simulink model "TxSteering_RxMVDR_4x4_HDL_IQ"  (R2020a)
settings: Solver=FixedStepDiscrete  StartTime=0.0  StopTime=stoptime*0 + inf  RelTol=1e-3
PreLoadFcn:
  | load('iq_bus_obj.mat');
  | model_init
InitFcn:
  | model_init
model workspace (MAT data in the model file):
  socvcb : containers.Map (value not decoded)
values from neighbouring files (symbols this model uses):
  BackSubstitutePrototype = fi(0, matrixdivbacksub_dt)    [model_init.m]
  DataSampleRate = ConverterSampleRate/DecimInterpFactor    (= 245760000)    [model_init.m]
  fc = ConverterSampleRate/4    (= 491520000)    [model_init.m]
  FPGAClkRate = DataSampleRate/VectorSamplingFactor    (= 245760000)    [model_init.m]
  matrixDivDelay = NumberOfCORDICIterations*10 + 86    [model_init.m]
  movavg_bitshift = nextpow2(sqrt(windowSize))    [model_init.m]
  mvdrPipelineDelay = covMatDelay+movAvgDelay+matrixDivDelay+normResponseDelay    [model_init.m]
  NCO_bits = 14    [model_init.m]
  numArrayElements = 4    [model_init.m]
  NumberOfCORDICIterations = matrixdivin_dt.WordLength - 1    [model_init.m]
  S2MM_frame_size = FrameSize*4    (= 40000)    [host_io_init.m]    (also in model_init.m = 1000)
  windowSize = 1024    [model_init.m]
undefined symbols (not defined in the file or in its folder): Fo, Fs, N, physconst
libraries: hdlsllib x268, simulink x53, dspsolvers x1, embreciprocals x1, dsphdlsigops x1
(part 10 of 12)

== system TxSteering_RxMVDR_4x4_HDL_IQ/DUT/MVDR/Compute Weight Vector/Matrix Left Divide/CORDIC/4x4 Complex CORDIC Matrix Left Divide/Q'B, R 4x4 Complex CORDIC Systolic Array/Leading Complex Row Rotation - 2/Rotate first element to real/Q'B, R Row Rotations - Real/Same Datatype3 ==
  Data : Inport
  Reference : Inport  Port=2
  Data Type Duplicate : DataTypeDuplicate
  DataOut : Outport  VectorParamsAs1DForOutWhenUnconnected=off
  wires:
  Data/1 -> Data Type Duplicate/1, DataOut/1
  Reference/1 -> Data Type Duplicate/2

== system TxSteering_RxMVDR_4x4_HDL_IQ/DUT/MVDR/Compute Weight Vector/Matrix Left Divide/CORDIC/4x4 Complex CORDIC Matrix Left Divide/Q'B, R 4x4 Complex CORDIC Systolic Array/Leading Complex Row Rotation - 2/Rotate first element to real - 1/Q'B, R Row Rotations - Real/CORDIC Counter ==
  validIn : Inport
  Compare To Constant : simulink/Logic and Bit Operations/Compare To Constant  relop===  const=NumberOfCORDICIterations-1  OutDataTypeStr=boolean
  Compare To Zero : simulink/Logic and Bit Operations/Compare To Zero  relop=>  OutDataTypeStr=boolean
  HDL Counter1 : hdlsllib/Sources/HDL Counter  CountType=Count limited  CountInit=0  CountStep=1  CountMax=NumberOfCORDICIterations-1  CountFromType=Initial value  CountFrom=0  CountResetPort=off  CountLoadPort=off  CountEnbPort=on  CountDirPort=off  CountDataType=Unsigned  CountWordLen=nextpow2(NumberOfCORDICIterations)  CountFracLen=0  CountSampTime=1
  OR : Logic  Operator=OR  IconShape=distinctive  AllPortsSameDT=off  OutDataTypeStr=boolean
  SR_latch : Subsystem
  State Control : StateControl  StateControl=Synchronous
  ValidIn to Ready Logic : Subsystem
  count_is_positive : Outport  VectorParamsAs1DForOutWhenUnconnected=off
  count : Outport  Port=2  VectorParamsAs1DForOutWhenUnconnected=off
  last : Outport  Port=3  VectorParamsAs1DForOutWhenUnconnected=off
  ready : Outport  Port=4  VectorParamsAs1DForOutWhenUnconnected=off
  wires:
  HDL Counter1/1 -> Compare To Zero/1, count/1, Compare To Constant/1  "count"
  OR/1 -> HDL Counter1/1
  Compare To Zero/1 -> count_is_positive/1, OR/1
  Compare To Constant/1 -> SR_latch/1(S), last/1
  validIn/1 -> ValidIn to Ready Logic/2(validIn), SR_latch/2(R), OR/2
  SR_latch/1(Q) -> ValidIn to Ready Logic/1(readyIn)  "ready"
  ValidIn to Ready Logic/1(readyOut) -> ready/1

== system TxSteering_RxMVDR_4x4_HDL_IQ/DUT/MVDR/Compute Weight Vector/Matrix Left Divide/CORDIC/4x4 Complex CORDIC Matrix Left Divide/Q'B, R 4x4 Complex CORDIC Systolic Array/Leading Complex Row Rotation - 2/Rotate first element to real - 1/Q'B, R Row Rotations - Real/Same Datatype ==
  Data : Inport
  Reference : Inport  Port=2
  Data Type Duplicate : DataTypeDuplicate
  DataOut : Outport  VectorParamsAs1DForOutWhenUnconnected=off
  wires:
  Data/1 -> Data Type Duplicate/1, DataOut/1
  Reference/1 -> Data Type Duplicate/2

== system TxSteering_RxMVDR_4x4_HDL_IQ/DUT/MVDR/Compute Weight Vector/Matrix Left Divide/CORDIC/4x4 Complex CORDIC Matrix Left Divide/Q'B, R 4x4 Complex CORDIC Systolic Array/Leading Complex Row Rotation - 2/Rotate first element to real - 1/Q'B, R Row Rotations - Real/Same Datatype1 ==
  Data : Inport
  Reference : Inport  Port=2
  Data Type Duplicate : DataTypeDuplicate
  DataOut : Outport  VectorParamsAs1DForOutWhenUnconnected=off
  wires:
  Data/1 -> Data Type Duplicate/1, DataOut/1
  Reference/1 -> Data Type Duplicate/2

== system TxSteering_RxMVDR_4x4_HDL_IQ/DUT/MVDR/Compute Weight Vector/Matrix Left Divide/CORDIC/4x4 Complex CORDIC Matrix Left Divide/Q'B, R 4x4 Complex CORDIC Systolic Array/Leading Complex Row Rotation - 2/Rotate first element to real - 1/Q'B, R Row Rotations - Real/Same Datatype2 ==
  Data : Inport
  Reference : Inport  Port=2
  Data Type Duplicate : DataTypeDuplicate
  DataOut : Outport  VectorParamsAs1DForOutWhenUnconnected=off
  wires:
  Data/1 -> Data Type Duplicate/1, DataOut/1
  Reference/1 -> Data Type Duplicate/2

== system TxSteering_RxMVDR_4x4_HDL_IQ/DUT/MVDR/Compute Weight Vector/Matrix Left Divide/CORDIC/4x4 Complex CORDIC Matrix Left Divide/Q'B, R 4x4 Complex CORDIC Systolic Array/Leading Complex Row Rotation - 2/Rotate first element to real - 1/Q'B, R Row Rotations - Real/Same Datatype3 ==
  Data : Inport
  Reference : Inport  Port=2
  Data Type Duplicate : DataTypeDuplicate
  DataOut : Outport  VectorParamsAs1DForOutWhenUnconnected=off
  wires:
  Data/1 -> Data Type Duplicate/1, DataOut/1
  Reference/1 -> Data Type Duplicate/2

== system TxSteering_RxMVDR_4x4_HDL_IQ/DUT/MVDR/Compute Weight Vector/Matrix Left Divide/CORDIC/4x4 Complex CORDIC Matrix Left Divide/Q'B, R 4x4 Complex CORDIC Systolic Array/Leading Complex Row Rotation - 3/Q'B, R Row Rotations - Complex/CORDIC Counter/SR_latch ==
  S : Inport
  R : Inport  Port=2
  AND : Logic  IconShape=distinctive  AllPortsSameDT=off  OutDataTypeStr=boolean
  NOT : Logic  Operator=NOT  IconShape=distinctive  AllPortsSameDT=off  OutDataTypeStr=boolean
  OR : Logic  Operator=OR  IconShape=distinctive  AllPortsSameDT=off  OutDataTypeStr=boolean
  Prev : UnitDelay  InitialCondition=1  SampleTime=-1  HasFrameUpgradeWarning=on
  Q : Outport  VectorParamsAs1DForOutWhenUnconnected=off
  wires:
  R/1 -> NOT/1
  NOT/1 -> AND/1
  AND/1 -> OR/2
  Prev/1 -> Q/1, AND/2
  OR/1 -> Prev/1
  S/1 -> OR/1

== system TxSteering_RxMVDR_4x4_HDL_IQ/DUT/MVDR/Compute Weight Vector/Matrix Left Divide/CORDIC/4x4 Complex CORDIC Matrix Left Divide/Q'B, R 4x4 Complex CORDIC Systolic Array/Leading Complex Row Rotation - 3/Q'B, R Row Rotations - Complex/CORDIC Counter/ValidIn to Ready Logic ==
  readyIn : Inport
  validIn : Inport  Port=2
  AND : Logic  IconShape=distinctive  AllPortsSameDT=off  OutDataTypeStr=boolean
  NOT : Logic  Operator=NOT  IconShape=distinctive  AllPortsSameDT=off  OutDataTypeStr=boolean
  readyOut : Outport  VectorParamsAs1DForOutWhenUnconnected=off
  wires:
  validIn/1 -> NOT/1
  readyIn/1 -> AND/1
  AND/1 -> readyOut/1
  NOT/1 -> AND/2

== system TxSteering_RxMVDR_4x4_HDL_IQ/DUT/MVDR/Compute Weight Vector/Matrix Left Divide/CORDIC/4x4 Complex CORDIC Matrix Left Divide/Q'B, R 4x4 Complex CORDIC Systolic Array/Leading Complex Row Rotation - 3/Rotate first element to real/Q'B, R Row Rotations - Real/CORDIC Counter ==
  validIn : Inport
  Compare To Constant : simulink/Logic and Bit Operations/Compare To Constant  relop===  const=NumberOfCORDICIterations-1  OutDataTypeStr=boolean
  Compare To Zero : simulink/Logic and Bit Operations/Compare To Zero  relop=>  OutDataTypeStr=boolean
  HDL Counter1 : hdlsllib/Sources/HDL Counter  CountType=Count limited  CountInit=0  CountStep=1  CountMax=NumberOfCORDICIterations-1  CountFromType=Initial value  CountFrom=0  CountResetPort=off  CountLoadPort=off  CountEnbPort=on  CountDirPort=off  CountDataType=Unsigned  CountWordLen=nextpow2(NumberOfCORDICIterations)  CountFracLen=0  CountSampTime=1
  OR : Logic  Operator=OR  IconShape=distinctive  AllPortsSameDT=off  OutDataTypeStr=boolean
  SR_latch : Subsystem
  State Control : StateControl  StateControl=Synchronous
  ValidIn to Ready Logic : Subsystem
  count_is_positive : Outport  VectorParamsAs1DForOutWhenUnconnected=off
  count : Outport  Port=2  VectorParamsAs1DForOutWhenUnconnected=off
  last : Outport  Port=3  VectorParamsAs1DForOutWhenUnconnected=off
  ready : Outport  Port=4  VectorParamsAs1DForOutWhenUnconnected=off
  wires:
  HDL Counter1/1 -> Compare To Zero/1, count/1, Compare To Constant/1  "count"
  OR/1 -> HDL Counter1/1
  Compare To Zero/1 -> count_is_positive/1, OR/1
  Compare To Constant/1 -> SR_latch/1(S), last/1
  validIn/1 -> ValidIn to Ready Logic/2(validIn), SR_latch/2(R), OR/2
  SR_latch/1(Q) -> ValidIn to Ready Logic/1(readyIn)  "ready"
  ValidIn to Ready Logic/1(readyOut) -> ready/1

== system TxSteering_RxMVDR_4x4_HDL_IQ/DUT/MVDR/Compute Weight Vector/Matrix Left Divide/CORDIC/4x4 Complex CORDIC Matrix Left Divide/Q'B, R 4x4 Complex CORDIC Systolic Array/Leading Complex Row Rotation - 3/Rotate first element to real/Q'B, R Row Rotations - Real/Same Datatype ==
  Data : Inport
  Reference : Inport  Port=2
  Data Type Duplicate : DataTypeDuplicate
  DataOut : Outport  VectorParamsAs1DForOutWhenUnconnected=off
  wires:
  Data/1 -> Data Type Duplicate/1, DataOut/1
  Reference/1 -> Data Type Duplicate/2

== system TxSteering_RxMVDR_4x4_HDL_IQ/DUT/MVDR/Compute Weight Vector/Matrix Left Divide/CORDIC/4x4 Complex CORDIC Matrix Left Divide/Q'B, R 4x4 Complex CORDIC Systolic Array/Leading Complex Row Rotation - 3/Rotate first element to real/Q'B, R Row Rotations - Real/Same Datatype1 ==
  Data : Inport
  Reference : Inport  Port=2
  Data Type Duplicate : DataTypeDuplicate
  DataOut : Outport  VectorParamsAs1DForOutWhenUnconnected=off
  wires:
  Data/1 -> Data Type Duplicate/1, DataOut/1
  Reference/1 -> Data Type Duplicate/2

== system TxSteering_RxMVDR_4x4_HDL_IQ/DUT/MVDR/Compute Weight Vector/Matrix Left Divide/CORDIC/4x4 Complex CORDIC Matrix Left Divide/Q'B, R 4x4 Complex CORDIC Systolic Array/Leading Complex Row Rotation - 3/Rotate first element to real/Q'B, R Row Rotations - Real/Same Datatype2 ==
  Data : Inport
  Reference : Inport  Port=2
  Data Type Duplicate : DataTypeDuplicate
  DataOut : Outport  VectorParamsAs1DForOutWhenUnconnected=off
  wires:
  Data/1 -> Data Type Duplicate/1, DataOut/1
  Reference/1 -> Data Type Duplicate/2

== system TxSteering_RxMVDR_4x4_HDL_IQ/DUT/MVDR/Compute Weight Vector/Matrix Left Divide/CORDIC/4x4 Complex CORDIC Matrix Left Divide/Q'B, R 4x4 Complex CORDIC Systolic Array/Leading Complex Row Rotation - 3/Rotate first element to real/Q'B, R Row Rotations - Real/Same Datatype3 ==
  Data : Inport
  Reference : Inport  Port=2
  Data Type Duplicate : DataTypeDuplicate
  DataOut : Outport  VectorParamsAs1DForOutWhenUnconnected=off
  wires:
  Data/1 -> Data Type Duplicate/1, DataOut/1
  Reference/1 -> Data Type Duplicate/2

== system TxSteering_RxMVDR_4x4_HDL_IQ/DUT/MVDR/Compute Weight Vector/Matrix Left Divide/CORDIC/4x4 Complex CORDIC Matrix Left Divide/Q'B, R 4x4 Complex CORDIC Systolic Array/Leading Complex Row Rotation - 3/Rotate first element to real - 1/Q'B, R Row Rotations - Real/CORDIC Counter ==
  validIn : Inport
  Compare To Constant : simulink/Logic and Bit Operations/Compare To Constant  relop===  const=NumberOfCORDICIterations-1  OutDataTypeStr=boolean
  Compare To Zero : simulink/Logic and Bit Operations/Compare To Zero  relop=>  OutDataTypeStr=boolean
  HDL Counter1 : hdlsllib/Sources/HDL Counter  CountType=Count limited  CountInit=0  CountStep=1  CountMax=NumberOfCORDICIterations-1  CountFromType=Initial value  CountFrom=0  CountResetPort=off  CountLoadPort=off  CountEnbPort=on  CountDirPort=off  CountDataType=Unsigned  CountWordLen=nextpow2(NumberOfCORDICIterations)  CountFracLen=0  CountSampTime=1
  OR : Logic  Operator=OR  IconShape=distinctive  AllPortsSameDT=off  OutDataTypeStr=boolean
  SR_latch : Subsystem
  State Control : StateControl  StateControl=Synchronous
  ValidIn to Ready Logic : Subsystem
  count_is_positive : Outport  VectorParamsAs1DForOutWhenUnconnected=off
  count : Outport  Port=2  VectorParamsAs1DForOutWhenUnconnected=off
  last : Outport  Port=3  VectorParamsAs1DForOutWhenUnconnected=off
  ready : Outport  Port=4  VectorParamsAs1DForOutWhenUnconnected=off
  wires:
  ValidIn to Ready Logic/1(readyOut) -> ready/1
  SR_latch/1(Q) -> ValidIn to Ready Logic/1(readyIn)  "ready"
  validIn/1 -> OR/2, SR_latch/2(R), ValidIn to Ready Logic/2(validIn)
  Compare To Constant/1 -> last/1, SR_latch/1(S)
  Compare To Zero/1 -> OR/1, count_is_positive/1
  OR/1 -> HDL Counter1/1
  HDL Counter1/1 -> Compare To Constant/1, count/1, Compare To Zero/1  "count"

== system TxSteering_RxMVDR_4x4_HDL_IQ/DUT/MVDR/Compute Weight Vector/Matrix Left Divide/CORDIC/4x4 Complex CORDIC Matrix Left Divide/Q'B, R 4x4 Complex CORDIC Systolic Array/Leading Complex Row Rotation - 3/Rotate first element to real - 1/Q'B, R Row Rotations - Real/Same Datatype ==
  Data : Inport
  Reference : Inport  Port=2
  Data Type Duplicate : DataTypeDuplicate
  DataOut : Outport  VectorParamsAs1DForOutWhenUnconnected=off
  wires:
  Data/1 -> Data Type Duplicate/1, DataOut/1
  Reference/1 -> Data Type Duplicate/2

== system TxSteering_RxMVDR_4x4_HDL_IQ/DUT/MVDR/Compute Weight Vector/Matrix Left Divide/CORDIC/4x4 Complex CORDIC Matrix Left Divide/Q'B, R 4x4 Complex CORDIC Systolic Array/Leading Complex Row Rotation - 3/Rotate first element to real - 1/Q'B, R Row Rotations - Real/Same Datatype1 ==
  Data : Inport
  Reference : Inport  Port=2
  Data Type Duplicate : DataTypeDuplicate
  DataOut : Outport  VectorParamsAs1DForOutWhenUnconnected=off
  wires:
  Data/1 -> Data Type Duplicate/1, DataOut/1
  Reference/1 -> Data Type Duplicate/2

== system TxSteering_RxMVDR_4x4_HDL_IQ/DUT/MVDR/Compute Weight Vector/Matrix Left Divide/CORDIC/4x4 Complex CORDIC Matrix Left Divide/Q'B, R 4x4 Complex CORDIC Systolic Array/Leading Complex Row Rotation - 3/Rotate first element to real - 1/Q'B, R Row Rotations - Real/Same Datatype2 ==
  Data : Inport
  Reference : Inport  Port=2
  Data Type Duplicate : DataTypeDuplicate
  DataOut : Outport  VectorParamsAs1DForOutWhenUnconnected=off
  wires:
  Data/1 -> Data Type Duplicate/1, DataOut/1
  Reference/1 -> Data Type Duplicate/2

== system TxSteering_RxMVDR_4x4_HDL_IQ/DUT/MVDR/Compute Weight Vector/Matrix Left Divide/CORDIC/4x4 Complex CORDIC Matrix Left Divide/Q'B, R 4x4 Complex CORDIC Systolic Array/Leading Complex Row Rotation - 3/Rotate first element to real - 1/Q'B, R Row Rotations - Real/Same Datatype3 ==
  Data : Inport
  Reference : Inport  Port=2
  Data Type Duplicate : DataTypeDuplicate
  DataOut : Outport  VectorParamsAs1DForOutWhenUnconnected=off
  wires:
  Data/1 -> Data Type Duplicate/1, DataOut/1
  Reference/1 -> Data Type Duplicate/2

== system TxSteering_RxMVDR_4x4_HDL_IQ/DUT/MVDR/Compute Weight Vector/Matrix Left Divide/CORDIC/4x4 Complex CORDIC Matrix Left Divide/Q'B, R 4x4 Complex CORDIC Systolic Array/Leading Complex Row Rotation - 4/Q'B, R Row Rotations - Complex/CORDIC Counter/SR_latch ==
  S : Inport
  R : Inport  Port=2
  AND : Logic  IconShape=distinctive  AllPortsSameDT=off  OutDataTypeStr=boolean
  NOT : Logic  Operator=NOT  IconShape=distinctive  AllPortsSameDT=off  OutDataTypeStr=boolean
  OR : Logic  Operator=OR  IconShape=distinctive  AllPortsSameDT=off  OutDataTypeStr=boolean
  Prev : UnitDelay  InitialCondition=1  SampleTime=-1  HasFrameUpgradeWarning=on
  Q : Outport  VectorParamsAs1DForOutWhenUnconnected=off
  wires:
  R/1 -> NOT/1
  NOT/1 -> AND/1
  AND/1 -> OR/2
  Prev/1 -> Q/1, AND/2
  OR/1 -> Prev/1
  S/1 -> OR/1

== system TxSteering_RxMVDR_4x4_HDL_IQ/DUT/MVDR/Compute Weight Vector/Matrix Left Divide/CORDIC/4x4 Complex CORDIC Matrix Left Divide/Q'B, R 4x4 Complex CORDIC Systolic Array/Leading Complex Row Rotation - 4/Q'B, R Row Rotations - Complex/CORDIC Counter/ValidIn to Ready Logic ==
  readyIn : Inport
  validIn : Inport  Port=2
  AND : Logic  IconShape=distinctive  AllPortsSameDT=off  OutDataTypeStr=boolean
  NOT : Logic  Operator=NOT  IconShape=distinctive  AllPortsSameDT=off  OutDataTypeStr=boolean
  readyOut : Outport  VectorParamsAs1DForOutWhenUnconnected=off
  wires:
  validIn/1 -> NOT/1
  readyIn/1 -> AND/1
  AND/1 -> readyOut/1
  NOT/1 -> AND/2

== system TxSteering_RxMVDR_4x4_HDL_IQ/DUT/MVDR/Compute Weight Vector/Matrix Left Divide/CORDIC/4x4 Complex CORDIC Matrix Left Divide/Q'B, R 4x4 Complex CORDIC Systolic Array/Leading Complex Row Rotation - 4/Rotate first element to real/Q'B, R Row Rotations - Real/CORDIC Counter ==
  validIn : Inport
  Compare To Constant : simulink/Logic and Bit Operations/Compare To Constant  relop===  const=NumberOfCORDICIterations-1  OutDataTypeStr=boolean
  Compare To Zero : simulink/Logic and Bit Operations/Compare To Zero  relop=>  OutDataTypeStr=boolean
  HDL Counter1 : hdlsllib/Sources/HDL Counter  CountType=Count limited  CountInit=0  CountStep=1  CountMax=NumberOfCORDICIterations-1  CountFromType=Initial value  CountFrom=0  CountResetPort=off  CountLoadPort=off  CountEnbPort=on  CountDirPort=off  CountDataType=Unsigned  CountWordLen=nextpow2(NumberOfCORDICIterations)  CountFracLen=0  CountSampTime=1
  OR : Logic  Operator=OR  IconShape=distinctive  AllPortsSameDT=off  OutDataTypeStr=boolean
  SR_latch : Subsystem
  State Control : StateControl  StateControl=Synchronous
  ValidIn to Ready Logic : Subsystem
  count_is_positive : Outport  VectorParamsAs1DForOutWhenUnconnected=off
  count : Outport  Port=2  VectorParamsAs1DForOutWhenUnconnected=off
  last : Outport  Port=3  VectorParamsAs1DForOutWhenUnconnected=off
  ready : Outport  Port=4  VectorParamsAs1DForOutWhenUnconnected=off
  wires:
  HDL Counter1/1 -> Compare To Zero/1, count/1, Compare To Constant/1  "count"
  OR/1 -> HDL Counter1/1
  Compare To Zero/1 -> count_is_positive/1, OR/1
  Compare To Constant/1 -> SR_latch/1(S), last/1
  validIn/1 -> ValidIn to Ready Logic/2(validIn), SR_latch/2(R), OR/2
  SR_latch/1(Q) -> ValidIn to Ready Logic/1(readyIn)  "ready"
  ValidIn to Ready Logic/1(readyOut) -> ready/1

== system TxSteering_RxMVDR_4x4_HDL_IQ/DUT/MVDR/Compute Weight Vector/Matrix Left Divide/CORDIC/4x4 Complex CORDIC Matrix Left Divide/Q'B, R 4x4 Complex CORDIC Systolic Array/Leading Complex Row Rotation - 4/Rotate first element to real/Q'B, R Row Rotations - Real/Same Datatype ==
  Data : Inport
  Reference : Inport  Port=2
  Data Type Duplicate : DataTypeDuplicate
  DataOut : Outport  VectorParamsAs1DForOutWhenUnconnected=off
  wires:
  Data/1 -> Data Type Duplicate/1, DataOut/1
  Reference/1 -> Data Type Duplicate/2

== system TxSteering_RxMVDR_4x4_HDL_IQ/DUT/MVDR/Compute Weight Vector/Matrix Left Divide/CORDIC/4x4 Complex CORDIC Matrix Left Divide/Q'B, R 4x4 Complex CORDIC Systolic Array/Leading Complex Row Rotation - 4/Rotate first element to real/Q'B, R Row Rotations - Real/Same Datatype1 ==
  Data : Inport
  Reference : Inport  Port=2
  Data Type Duplicate : DataTypeDuplicate
  DataOut : Outport  VectorParamsAs1DForOutWhenUnconnected=off
  wires:
  Data/1 -> Data Type Duplicate/1, DataOut/1
  Reference/1 -> Data Type Duplicate/2

== system TxSteering_RxMVDR_4x4_HDL_IQ/DUT/MVDR/Compute Weight Vector/Matrix Left Divide/CORDIC/4x4 Complex CORDIC Matrix Left Divide/Q'B, R 4x4 Complex CORDIC Systolic Array/Leading Complex Row Rotation - 4/Rotate first element to real/Q'B, R Row Rotations - Real/Same Datatype2 ==
  Data : Inport
  Reference : Inport  Port=2
  Data Type Duplicate : DataTypeDuplicate
  DataOut : Outport  VectorParamsAs1DForOutWhenUnconnected=off
  wires:
  Data/1 -> Data Type Duplicate/1, DataOut/1
  Reference/1 -> Data Type Duplicate/2

== system TxSteering_RxMVDR_4x4_HDL_IQ/DUT/MVDR/Compute Weight Vector/Matrix Left Divide/CORDIC/4x4 Complex CORDIC Matrix Left Divide/Q'B, R 4x4 Complex CORDIC Systolic Array/Leading Complex Row Rotation - 4/Rotate first element to real/Q'B, R Row Rotations - Real/Same Datatype3 ==
  Data : Inport
  Reference : Inport  Port=2
  Data Type Duplicate : DataTypeDuplicate
  DataOut : Outport  VectorParamsAs1DForOutWhenUnconnected=off
  wires:
  Data/1 -> Data Type Duplicate/1, DataOut/1
  Reference/1 -> Data Type Duplicate/2

== system TxSteering_RxMVDR_4x4_HDL_IQ/DUT/MVDR/Compute Weight Vector/Matrix Left Divide/CORDIC/4x4 Complex CORDIC Matrix Left Divide/Q'B, R 4x4 Complex CORDIC Systolic Array/Leading Complex Row Rotation - 4/Rotate first element to real - 1/Q'B, R Row Rotations - Real/CORDIC Counter ==
  validIn : Inport
  Compare To Constant : simulink/Logic and Bit Operations/Compare To Constant  relop===  const=NumberOfCORDICIterations-1  OutDataTypeStr=boolean
  Compare To Zero : simulink/Logic and Bit Operations/Compare To Zero  relop=>  OutDataTypeStr=boolean
  HDL Counter1 : hdlsllib/Sources/HDL Counter  CountType=Count limited  CountInit=0  CountStep=1  CountMax=NumberOfCORDICIterations-1  CountFromType=Initial value  CountFrom=0  CountResetPort=off  CountLoadPort=off  CountEnbPort=on  CountDirPort=off  CountDataType=Unsigned  CountWordLen=nextpow2(NumberOfCORDICIterations)  CountFracLen=0  CountSampTime=1
  OR : Logic  Operator=OR  IconShape=distinctive  AllPortsSameDT=off  OutDataTypeStr=boolean
  SR_latch : Subsystem
  State Control : StateControl  StateControl=Synchronous
  ValidIn to Ready Logic : Subsystem
  count_is_positive : Outport  VectorParamsAs1DForOutWhenUnconnected=off
  count : Outport  Port=2  VectorParamsAs1DForOutWhenUnconnected=off
  last : Outport  Port=3  VectorParamsAs1DForOutWhenUnconnected=off
  ready : Outport  Port=4  VectorParamsAs1DForOutWhenUnconnected=off
  wires:
  ValidIn to Ready Logic/1(readyOut) -> ready/1
  SR_latch/1(Q) -> ValidIn to Ready Logic/1(readyIn)  "ready"
  validIn/1 -> OR/2, SR_latch/2(R), ValidIn to Ready Logic/2(validIn)
  Compare To Constant/1 -> last/1, SR_latch/1(S)
  Compare To Zero/1 -> OR/1, count_is_positive/1
  OR/1 -> HDL Counter1/1
  HDL Counter1/1 -> Compare To Constant/1, count/1, Compare To Zero/1  "count"

== system TxSteering_RxMVDR_4x4_HDL_IQ/DUT/MVDR/Compute Weight Vector/Matrix Left Divide/CORDIC/4x4 Complex CORDIC Matrix Left Divide/Q'B, R 4x4 Complex CORDIC Systolic Array/Leading Complex Row Rotation - 4/Rotate first element to real - 1/Q'B, R Row Rotations - Real/Same Datatype ==
  Data : Inport
  Reference : Inport  Port=2
  Data Type Duplicate : DataTypeDuplicate
  DataOut : Outport  VectorParamsAs1DForOutWhenUnconnected=off
  wires:
  Data/1 -> Data Type Duplicate/1, DataOut/1
  Reference/1 -> Data Type Duplicate/2

== system TxSteering_RxMVDR_4x4_HDL_IQ/DUT/MVDR/Compute Weight Vector/Matrix Left Divide/CORDIC/4x4 Complex CORDIC Matrix Left Divide/Q'B, R 4x4 Complex CORDIC Systolic Array/Leading Complex Row Rotation - 4/Rotate first element to real - 1/Q'B, R Row Rotations - Real/Same Datatype1 ==
  Data : Inport
  Reference : Inport  Port=2
  Data Type Duplicate : DataTypeDuplicate
  DataOut : Outport  VectorParamsAs1DForOutWhenUnconnected=off
  wires:
  Data/1 -> Data Type Duplicate/1, DataOut/1
  Reference/1 -> Data Type Duplicate/2

== system TxSteering_RxMVDR_4x4_HDL_IQ/DUT/MVDR/Compute Weight Vector/Matrix Left Divide/CORDIC/4x4 Complex CORDIC Matrix Left Divide/Q'B, R 4x4 Complex CORDIC Systolic Array/Leading Complex Row Rotation - 4/Rotate first element to real - 1/Q'B, R Row Rotations - Real/Same Datatype2 ==
  Data : Inport
  Reference : Inport  Port=2
  Data Type Duplicate : DataTypeDuplicate
  DataOut : Outport  VectorParamsAs1DForOutWhenUnconnected=off
  wires:
  Data/1 -> Data Type Duplicate/1, DataOut/1
  Reference/1 -> Data Type Duplicate/2

== system TxSteering_RxMVDR_4x4_HDL_IQ/DUT/MVDR/Compute Weight Vector/Matrix Left Divide/CORDIC/4x4 Complex CORDIC Matrix Left Divide/Q'B, R 4x4 Complex CORDIC Systolic Array/Leading Complex Row Rotation - 4/Rotate first element to real - 1/Q'B, R Row Rotations - Real/Same Datatype3 ==
  Data : Inport
  Reference : Inport  Port=2
  Data Type Duplicate : DataTypeDuplicate
  DataOut : Outport  VectorParamsAs1DForOutWhenUnconnected=off
  wires:
  Data/1 -> Data Type Duplicate/1, DataOut/1
  Reference/1 -> Data Type Duplicate/2

== system TxSteering_RxMVDR_4x4_HDL_IQ/DUT/MVDR/Compute Weight Vector/Matrix Left Divide/CORDIC/4x4 Complex CORDIC Matrix Left Divide/Q'B, R 4x4 Complex CORDIC Systolic Array/Rotate first element to real/Q'B, R Row Rotations - Real/CORDIC Counter/SR_latch ==
  S : Inport
  R : Inport  Port=2
  AND : Logic  IconShape=distinctive  AllPortsSameDT=off  OutDataTypeStr=boolean
  NOT : Logic  Operator=NOT  IconShape=distinctive  AllPortsSameDT=off  OutDataTypeStr=boolean
  OR : Logic  Operator=OR  IconShape=distinctive  AllPortsSameDT=off  OutDataTypeStr=boolean
  Prev : UnitDelay  InitialCondition=1  SampleTime=-1  HasFrameUpgradeWarning=on
  Q : Outport  VectorParamsAs1DForOutWhenUnconnected=off
  wires:
  R/1 -> NOT/1
  NOT/1 -> AND/1
  AND/1 -> OR/2
  Prev/1 -> Q/1, AND/2
  OR/1 -> Prev/1
  S/1 -> OR/1

== system TxSteering_RxMVDR_4x4_HDL_IQ/DUT/MVDR/Compute Weight Vector/Matrix Left Divide/CORDIC/4x4 Complex CORDIC Matrix Left Divide/Q'B, R 4x4 Complex CORDIC Systolic Array/Rotate first element to real/Q'B, R Row Rotations - Real/CORDIC Counter/ValidIn to Ready Logic ==
  readyIn : Inport
  validIn : Inport  Port=2
  AND : Logic  IconShape=distinctive  AllPortsSameDT=off  OutDataTypeStr=boolean
  NOT : Logic  Operator=NOT  IconShape=distinctive  AllPortsSameDT=off  OutDataTypeStr=boolean
  readyOut : Outport  VectorParamsAs1DForOutWhenUnconnected=off
  wires:
  validIn/1 -> NOT/1
  readyIn/1 -> AND/1
  AND/1 -> readyOut/1
  NOT/1 -> AND/2

== system TxSteering_RxMVDR_4x4_HDL_IQ/DUT/MVDR/Compute Weight Vector/Matrix Left Divide/CORDIC/4x4 Complex CORDIC Matrix Left Divide/Back Substitute 4x4 Complex CORDIC/Invert first element - Folded/CORDIC Reciprocal Normalized, Folded/CORDIC Reciprocal Rotations- Folded/CORDIC Counter/SR_latch ==
  S : Inport
  R : Inport  Port=2
  AND : Logic  IconShape=distinctive  AllPortsSameDT=off  OutDataTypeStr=boolean
  NOT : Logic  Operator=NOT  IconShape=distinctive  AllPortsSameDT=off  OutDataTypeStr=boolean
  OR : Logic  Operator=OR  IconShape=distinctive  AllPortsSameDT=off  OutDataTypeStr=boolean
  Prev : UnitDelay  InitialCondition=1  SampleTime=-1  HasFrameUpgradeWarning=on
  Q : Outport  VectorParamsAs1DForOutWhenUnconnected=off
  wires:
  S/1 -> OR/1
  OR/1 -> Prev/1
  Prev/1 -> AND/2, Q/1
  AND/1 -> OR/2
  NOT/1 -> AND/1
  R/1 -> NOT/1

== system TxSteering_RxMVDR_4x4_HDL_IQ/DUT/MVDR/Compute Weight Vector/Matrix Left Divide/CORDIC/4x4 Complex CORDIC Matrix Left Divide/Back Substitute 4x4 Complex CORDIC/Invert first element - Folded/CORDIC Reciprocal Normalized, Folded/CORDIC Reciprocal Rotations- Folded/CORDIC Counter/ValidIn to Ready Logic ==
  readyIn : Inport
  validIn : Inport  Port=2
  AND : Logic  IconShape=distinctive  AllPortsSameDT=off  OutDataTypeStr=boolean
  NOT : Logic  Operator=NOT  IconShape=distinctive  AllPortsSameDT=off  OutDataTypeStr=boolean
  readyOut : Outport  VectorParamsAs1DForOutWhenUnconnected=off
  wires:
  validIn/1 -> NOT/1
  readyIn/1 -> AND/1
  AND/1 -> readyOut/1
  NOT/1 -> AND/2

== system TxSteering_RxMVDR_4x4_HDL_IQ/DUT/MVDR/Compute Weight Vector/Matrix Left Divide/CORDIC/4x4 Complex CORDIC Matrix Left Divide/Back Substitute 4x4 Complex CORDIC/Invert first element - Folded1/CORDIC Reciprocal Normalized, Folded/CORDIC Reciprocal Rotations- Folded/CORDIC Counter/SR_latch ==
  S : Inport
  R : Inport  Port=2
  AND : Logic  IconShape=distinctive  AllPortsSameDT=off  OutDataTypeStr=boolean
  NOT : Logic  Operator=NOT  IconShape=distinctive  AllPortsSameDT=off  OutDataTypeStr=boolean
  OR : Logic  Operator=OR  IconShape=distinctive  AllPortsSameDT=off  OutDataTypeStr=boolean
  Prev : UnitDelay  InitialCondition=1  SampleTime=-1  HasFrameUpgradeWarning=on
  Q : Outport  VectorParamsAs1DForOutWhenUnconnected=off
  wires:
  R/1 -> NOT/1
  NOT/1 -> AND/1
  AND/1 -> OR/2
  Prev/1 -> Q/1, AND/2
  OR/1 -> Prev/1
  S/1 -> OR/1

== system TxSteering_RxMVDR_4x4_HDL_IQ/DUT/MVDR/Compute Weight Vector/Matrix Left Divide/CORDIC/4x4 Complex CORDIC Matrix Left Divide/Back Substitute 4x4 Complex CORDIC/Invert first element - Folded1/CORDIC Reciprocal Normalized, Folded/CORDIC Reciprocal Rotations- Folded/CORDIC Counter/ValidIn to Ready Logic ==
  readyIn : Inport
  validIn : Inport  Port=2
  AND : Logic  IconShape=distinctive  AllPortsSameDT=off  OutDataTypeStr=boolean
  NOT : Logic  Operator=NOT  IconShape=distinctive  AllPortsSameDT=off  OutDataTypeStr=boolean
  readyOut : Outport  VectorParamsAs1DForOutWhenUnconnected=off
  wires:
  validIn/1 -> NOT/1
  readyIn/1 -> AND/1
  AND/1 -> readyOut/1
  NOT/1 -> AND/2

== system TxSteering_RxMVDR_4x4_HDL_IQ/DUT/MVDR/Compute Weight Vector/Matrix Left Divide/CORDIC/4x4 Complex CORDIC Matrix Left Divide/Back Substitute 4x4 Complex CORDIC/Invert first element - Folded2/CORDIC Reciprocal Normalized, Folded/CORDIC Reciprocal Rotations- Folded/CORDIC Counter/SR_latch ==
  S : Inport
  R : Inport  Port=2
  AND : Logic  IconShape=distinctive  AllPortsSameDT=off  OutDataTypeStr=boolean
  NOT : Logic  Operator=NOT  IconShape=distinctive  AllPortsSameDT=off  OutDataTypeStr=boolean
  OR : Logic  Operator=OR  IconShape=distinctive  AllPortsSameDT=off  OutDataTypeStr=boolean
  Prev : UnitDelay  InitialCondition=1  SampleTime=-1  HasFrameUpgradeWarning=on
  Q : Outport  VectorParamsAs1DForOutWhenUnconnected=off
  wires:
  R/1 -> NOT/1
  NOT/1 -> AND/1
  AND/1 -> OR/2
  Prev/1 -> Q/1, AND/2
  OR/1 -> Prev/1
  S/1 -> OR/1

== system TxSteering_RxMVDR_4x4_HDL_IQ/DUT/MVDR/Compute Weight Vector/Matrix Left Divide/CORDIC/4x4 Complex CORDIC Matrix Left Divide/Back Substitute 4x4 Complex CORDIC/Invert first element - Folded2/CORDIC Reciprocal Normalized, Folded/CORDIC Reciprocal Rotations- Folded/CORDIC Counter/ValidIn to Ready Logic ==
  readyIn : Inport
  validIn : Inport  Port=2
  AND : Logic  IconShape=distinctive  AllPortsSameDT=off  OutDataTypeStr=boolean
  NOT : Logic  Operator=NOT  IconShape=distinctive  AllPortsSameDT=off  OutDataTypeStr=boolean
  readyOut : Outport  VectorParamsAs1DForOutWhenUnconnected=off
  wires:
  validIn/1 -> NOT/1
  readyIn/1 -> AND/1
  AND/1 -> readyOut/1
  NOT/1 -> AND/2

== system TxSteering_RxMVDR_4x4_HDL_IQ/DUT/MVDR/Compute Weight Vector/Matrix Left Divide/CORDIC/4x4 Complex CORDIC Matrix Left Divide/Back Substitute 4x4 Complex CORDIC/Invert first element - Folded3/CORDIC Reciprocal Normalized, Folded/CORDIC Reciprocal Rotations- Folded/CORDIC Counter/SR_latch ==
  S : Inport
  R : Inport  Port=2
  AND : Logic  IconShape=distinctive  AllPortsSameDT=off  OutDataTypeStr=boolean
  NOT : Logic  Operator=NOT  IconShape=distinctive  AllPortsSameDT=off  OutDataTypeStr=boolean
  OR : Logic  Operator=OR  IconShape=distinctive  AllPortsSameDT=off  OutDataTypeStr=boolean
  Prev : UnitDelay  InitialCondition=1  SampleTime=-1  HasFrameUpgradeWarning=on
  Q : Outport  VectorParamsAs1DForOutWhenUnconnected=off
  wires:
  R/1 -> NOT/1
  NOT/1 -> AND/1
  AND/1 -> OR/2
  Prev/1 -> Q/1, AND/2
  OR/1 -> Prev/1
  S/1 -> OR/1

== system TxSteering_RxMVDR_4x4_HDL_IQ/DUT/MVDR/Compute Weight Vector/Matrix Left Divide/CORDIC/4x4 Complex CORDIC Matrix Left Divide/Back Substitute 4x4 Complex CORDIC/Invert first element - Folded3/CORDIC Reciprocal Normalized, Folded/CORDIC Reciprocal Rotations- Folded/CORDIC Counter/ValidIn to Ready Logic ==
  readyIn : Inport
  validIn : Inport  Port=2
  AND : Logic  IconShape=distinctive  AllPortsSameDT=off  OutDataTypeStr=boolean
  NOT : Logic  Operator=NOT  IconShape=distinctive  AllPortsSameDT=off  OutDataTypeStr=boolean
  readyOut : Outport  VectorParamsAs1DForOutWhenUnconnected=off
  wires:
  validIn/1 -> NOT/1
  readyIn/1 -> AND/1
  AND/1 -> readyOut/1
  NOT/1 -> AND/2

== system TxSteering_RxMVDR_4x4_HDL_IQ/DUT/MVDR/Compute Weight Vector/Matrix Left Divide/CORDIC/4x4 Complex CORDIC Matrix Left Divide/Q'B, R 4x4 Complex CORDIC Systolic Array/Complex Row Rotation 1/Rotate first element to real - Folded/Q'B, R Row Rotations - Real/CORDIC Counter/SR_latch ==
  S : Inport
  R : Inport  Port=2
  AND : Logic  IconShape=distinctive  AllPortsSameDT=off  OutDataTypeStr=boolean
  NOT : Logic  Operator=NOT  IconShape=distinctive  AllPortsSameDT=off  OutDataTypeStr=boolean
  OR : Logic  Operator=OR  IconShape=distinctive  AllPortsSameDT=off  OutDataTypeStr=boolean
  Prev : UnitDelay  InitialCondition=1  SampleTime=-1  HasFrameUpgradeWarning=on
  Q : Outport  VectorParamsAs1DForOutWhenUnconnected=off
  wires:
  S/1 -> OR/1
  OR/1 -> Prev/1
  Prev/1 -> AND/2, Q/1
  AND/1 -> OR/2
  NOT/1 -> AND/1
  R/1 -> NOT/1

== system TxSteering_RxMVDR_4x4_HDL_IQ/DUT/MVDR/Compute Weight Vector/Matrix Left Divide/CORDIC/4x4 Complex CORDIC Matrix Left Divide/Q'B, R 4x4 Complex CORDIC Systolic Array/Complex Row Rotation 1/Rotate first element to real - Folded/Q'B, R Row Rotations - Real/CORDIC Counter/ValidIn to Ready Logic ==
  readyIn : Inport
  validIn : Inport  Port=2
  AND : Logic  IconShape=distinctive  AllPortsSameDT=off  OutDataTypeStr=boolean
  NOT : Logic  Operator=NOT  IconShape=distinctive  AllPortsSameDT=off  OutDataTypeStr=boolean
  readyOut : Outport  VectorParamsAs1DForOutWhenUnconnected=off
  wires:
  validIn/1 -> NOT/1
  readyIn/1 -> AND/1
  AND/1 -> readyOut/1
  NOT/1 -> AND/2

== system TxSteering_RxMVDR_4x4_HDL_IQ/DUT/MVDR/Compute Weight Vector/Matrix Left Divide/CORDIC/4x4 Complex CORDIC Matrix Left Divide/Q'B, R 4x4 Complex CORDIC Systolic Array/Leading Complex Row Rotation/Rotate first element to real/Q'B, R Row Rotations - Real/CORDIC Counter/SR_latch ==
  S : Inport
  R : Inport  Port=2
  AND : Logic  IconShape=distinctive  AllPortsSameDT=off  OutDataTypeStr=boolean
  NOT : Logic  Operator=NOT  IconShape=distinctive  AllPortsSameDT=off  OutDataTypeStr=boolean
  OR : Logic  Operator=OR  IconShape=distinctive  AllPortsSameDT=off  OutDataTypeStr=boolean
  Prev : UnitDelay  InitialCondition=1  SampleTime=-1  HasFrameUpgradeWarning=on
  Q : Outport  VectorParamsAs1DForOutWhenUnconnected=off
  wires:
  R/1 -> NOT/1
  NOT/1 -> AND/1
  AND/1 -> OR/2
  Prev/1 -> Q/1, AND/2
  OR/1 -> Prev/1
  S/1 -> OR/1

== system TxSteering_RxMVDR_4x4_HDL_IQ/DUT/MVDR/Compute Weight Vector/Matrix Left Divide/CORDIC/4x4 Complex CORDIC Matrix Left Divide/Q'B, R 4x4 Complex CORDIC Systolic Array/Leading Complex Row Rotation/Rotate first element to real/Q'B, R Row Rotations - Real/CORDIC Counter/ValidIn to Ready Logic ==
  readyIn : Inport
  validIn : Inport  Port=2
  AND : Logic  IconShape=distinctive  AllPortsSameDT=off  OutDataTypeStr=boolean
  NOT : Logic  Operator=NOT  IconShape=distinctive  AllPortsSameDT=off  OutDataTypeStr=boolean
  readyOut : Outport  VectorParamsAs1DForOutWhenUnconnected=off
  wires:
  validIn/1 -> NOT/1
  readyIn/1 -> AND/1
  AND/1 -> readyOut/1
  NOT/1 -> AND/2

== system TxSteering_RxMVDR_4x4_HDL_IQ/DUT/MVDR/Compute Weight Vector/Matrix Left Divide/CORDIC/4x4 Complex CORDIC Matrix Left Divide/Q'B, R 4x4 Complex CORDIC Systolic Array/Leading Complex Row Rotation/Rotate first element to real - 1/Q'B, R Row Rotations - Real/CORDIC Counter/SR_latch ==
  S : Inport
  R : Inport  Port=2
  AND : Logic  IconShape=distinctive  AllPortsSameDT=off  OutDataTypeStr=boolean
  NOT : Logic  Operator=NOT  IconShape=distinctive  AllPortsSameDT=off  OutDataTypeStr=boolean
  OR : Logic  Operator=OR  IconShape=distinctive  AllPortsSameDT=off  OutDataTypeStr=boolean
  Prev : UnitDelay  InitialCondition=1  SampleTime=-1  HasFrameUpgradeWarning=on
  Q : Outport  VectorParamsAs1DForOutWhenUnconnected=off
  wires:
  R/1 -> NOT/1
  NOT/1 -> AND/1
  AND/1 -> OR/2
  Prev/1 -> Q/1, AND/2
  OR/1 -> Prev/1
  S/1 -> OR/1

== system TxSteering_RxMVDR_4x4_HDL_IQ/DUT/MVDR/Compute Weight Vector/Matrix Left Divide/CORDIC/4x4 Complex CORDIC Matrix Left Divide/Q'B, R 4x4 Complex CORDIC Systolic Array/Leading Complex Row Rotation/Rotate first element to real - 1/Q'B, R Row Rotations - Real/CORDIC Counter/ValidIn to Ready Logic ==
  readyIn : Inport
  validIn : Inport  Port=2
  AND : Logic  IconShape=distinctive  AllPortsSameDT=off  OutDataTypeStr=boolean
  NOT : Logic  Operator=NOT  IconShape=distinctive  AllPortsSameDT=off  OutDataTypeStr=boolean
  readyOut : Outport  VectorParamsAs1DForOutWhenUnconnected=off
  wires:
  validIn/1 -> NOT/1
  readyIn/1 -> AND/1
  AND/1 -> readyOut/1
  NOT/1 -> AND/2

== system TxSteering_RxMVDR_4x4_HDL_IQ/DUT/MVDR/Compute Weight Vector/Matrix Left Divide/CORDIC/4x4 Complex CORDIC Matrix Left Divide/Q'B, R 4x4 Complex CORDIC Systolic Array/Leading Complex Row Rotation - 2/Rotate first element to real/Q'B, R Row Rotations - Real/CORDIC Counter/SR_latch ==
  S : Inport
  R : Inport  Port=2
  AND : Logic  IconShape=distinctive  AllPortsSameDT=off  OutDataTypeStr=boolean
  NOT : Logic  Operator=NOT  IconShape=distinctive  AllPortsSameDT=off  OutDataTypeStr=boolean
  OR : Logic  Operator=OR  IconShape=distinctive  AllPortsSameDT=off  OutDataTypeStr=boolean
  Prev : UnitDelay  InitialCondition=1  SampleTime=-1  HasFrameUpgradeWarning=on
  Q : Outport  VectorParamsAs1DForOutWhenUnconnected=off
  wires:
  R/1 -> NOT/1
  NOT/1 -> AND/1
  AND/1 -> OR/2
  Prev/1 -> Q/1, AND/2
  OR/1 -> Prev/1
  S/1 -> OR/1

== system TxSteering_RxMVDR_4x4_HDL_IQ/DUT/MVDR/Compute Weight Vector/Matrix Left Divide/CORDIC/4x4 Complex CORDIC Matrix Left Divide/Q'B, R 4x4 Complex CORDIC Systolic Array/Leading Complex Row Rotation - 2/Rotate first element to real/Q'B, R Row Rotations - Real/CORDIC Counter/ValidIn to Ready Logic ==
  readyIn : Inport
  validIn : Inport  Port=2
  AND : Logic  IconShape=distinctive  AllPortsSameDT=off  OutDataTypeStr=boolean
  NOT : Logic  Operator=NOT  IconShape=distinctive  AllPortsSameDT=off  OutDataTypeStr=boolean
  readyOut : Outport  VectorParamsAs1DForOutWhenUnconnected=off
  wires:
  validIn/1 -> NOT/1
  readyIn/1 -> AND/1
  AND/1 -> readyOut/1
  NOT/1 -> AND/2

== system TxSteering_RxMVDR_4x4_HDL_IQ/DUT/MVDR/Compute Weight Vector/Matrix Left Divide/CORDIC/4x4 Complex CORDIC Matrix Left Divide/Q'B, R 4x4 Complex CORDIC Systolic Array/Leading Complex Row Rotation - 2/Rotate first element to real - 1/Q'B, R Row Rotations - Real/CORDIC Counter/SR_latch ==
  S : Inport
  R : Inport  Port=2
  AND : Logic  IconShape=distinctive  AllPortsSameDT=off  OutDataTypeStr=boolean
  NOT : Logic  Operator=NOT  IconShape=distinctive  AllPortsSameDT=off  OutDataTypeStr=boolean
  OR : Logic  Operator=OR  IconShape=distinctive  AllPortsSameDT=off  OutDataTypeStr=boolean
  Prev : UnitDelay  InitialCondition=1  SampleTime=-1  HasFrameUpgradeWarning=on
  Q : Outport  VectorParamsAs1DForOutWhenUnconnected=off
  wires:
  S/1 -> OR/1
  OR/1 -> Prev/1
  Prev/1 -> AND/2, Q/1
  AND/1 -> OR/2
  NOT/1 -> AND/1
  R/1 -> NOT/1

== system TxSteering_RxMVDR_4x4_HDL_IQ/DUT/MVDR/Compute Weight Vector/Matrix Left Divide/CORDIC/4x4 Complex CORDIC Matrix Left Divide/Q'B, R 4x4 Complex CORDIC Systolic Array/Leading Complex Row Rotation - 2/Rotate first element to real - 1/Q'B, R Row Rotations - Real/CORDIC Counter/ValidIn to Ready Logic ==
  readyIn : Inport
  validIn : Inport  Port=2
  AND : Logic  IconShape=distinctive  AllPortsSameDT=off  OutDataTypeStr=boolean
  NOT : Logic  Operator=NOT  IconShape=distinctive  AllPortsSameDT=off  OutDataTypeStr=boolean
  readyOut : Outport  VectorParamsAs1DForOutWhenUnconnected=off
  wires:
  validIn/1 -> NOT/1
  readyIn/1 -> AND/1
  AND/1 -> readyOut/1
  NOT/1 -> AND/2

== system TxSteering_RxMVDR_4x4_HDL_IQ/DUT/MVDR/Compute Weight Vector/Matrix Left Divide/CORDIC/4x4 Complex CORDIC Matrix Left Divide/Q'B, R 4x4 Complex CORDIC Systolic Array/Leading Complex Row Rotation - 3/Rotate first element to real/Q'B, R Row Rotations - Real/CORDIC Counter/SR_latch ==
  S : Inport
  R : Inport  Port=2
  AND : Logic  IconShape=distinctive  AllPortsSameDT=off  OutDataTypeStr=boolean
  NOT : Logic  Operator=NOT  IconShape=distinctive  AllPortsSameDT=off  OutDataTypeStr=boolean
  OR : Logic  Operator=OR  IconShape=distinctive  AllPortsSameDT=off  OutDataTypeStr=boolean
  Prev : UnitDelay  InitialCondition=1  SampleTime=-1  HasFrameUpgradeWarning=on
  Q : Outport  VectorParamsAs1DForOutWhenUnconnected=off
  wires:
  S/1 -> OR/1
  OR/1 -> Prev/1
  Prev/1 -> AND/2, Q/1
  AND/1 -> OR/2
  NOT/1 -> AND/1
  R/1 -> NOT/1

== system TxSteering_RxMVDR_4x4_HDL_IQ/DUT/MVDR/Compute Weight Vector/Matrix Left Divide/CORDIC/4x4 Complex CORDIC Matrix Left Divide/Q'B, R 4x4 Complex CORDIC Systolic Array/Leading Complex Row Rotation - 3/Rotate first element to real/Q'B, R Row Rotations - Real/CORDIC Counter/ValidIn to Ready Logic ==
  readyIn : Inport
  validIn : Inport  Port=2
  AND : Logic  IconShape=distinctive  AllPortsSameDT=off  OutDataTypeStr=boolean
  NOT : Logic  Operator=NOT  IconShape=distinctive  AllPortsSameDT=off  OutDataTypeStr=boolean
  readyOut : Outport  VectorParamsAs1DForOutWhenUnconnected=off
  wires:
  validIn/1 -> NOT/1
  readyIn/1 -> AND/1
  AND/1 -> readyOut/1
  NOT/1 -> AND/2

== system TxSteering_RxMVDR_4x4_HDL_IQ/DUT/MVDR/Compute Weight Vector/Matrix Left Divide/CORDIC/4x4 Complex CORDIC Matrix Left Divide/Q'B, R 4x4 Complex CORDIC Systolic Array/Leading Complex Row Rotation - 3/Rotate first element to real - 1/Q'B, R Row Rotations - Real/CORDIC Counter/SR_latch ==
  S : Inport
  R : Inport  Port=2
  AND : Logic  IconShape=distinctive  AllPortsSameDT=off  OutDataTypeStr=boolean
  NOT : Logic  Operator=NOT  IconShape=distinctive  AllPortsSameDT=off  OutDataTypeStr=boolean
  OR : Logic  Operator=OR  IconShape=distinctive  AllPortsSameDT=off  OutDataTypeStr=boolean
  Prev : UnitDelay  InitialCondition=1  SampleTime=-1  HasFrameUpgradeWarning=on
  Q : Outport  VectorParamsAs1DForOutWhenUnconnected=off
  wires:
  R/1 -> NOT/1
  NOT/1 -> AND/1
  AND/1 -> OR/2
  Prev/1 -> Q/1, AND/2
  OR/1 -> Prev/1
  S/1 -> OR/1

== system TxSteering_RxMVDR_4x4_HDL_IQ/DUT/MVDR/Compute Weight Vector/Matrix Left Divide/CORDIC/4x4 Complex CORDIC Matrix Left Divide/Q'B, R 4x4 Complex CORDIC Systolic Array/Leading Complex Row Rotation - 3/Rotate first element to real - 1/Q'B, R Row Rotations - Real/CORDIC Counter/ValidIn to Ready Logic ==
  readyIn : Inport
  validIn : Inport  Port=2
  AND : Logic  IconShape=distinctive  AllPortsSameDT=off  OutDataTypeStr=boolean
  NOT : Logic  Operator=NOT  IconShape=distinctive  AllPortsSameDT=off  OutDataTypeStr=boolean
  readyOut : Outport  VectorParamsAs1DForOutWhenUnconnected=off
  wires:
  validIn/1 -> NOT/1
  readyIn/1 -> AND/1
  AND/1 -> readyOut/1
  NOT/1 -> AND/2

== system TxSteering_RxMVDR_4x4_HDL_IQ/DUT/MVDR/Compute Weight Vector/Matrix Left Divide/CORDIC/4x4 Complex CORDIC Matrix Left Divide/Q'B, R 4x4 Complex CORDIC Systolic Array/Leading Complex Row Rotation - 4/Rotate first element to real/Q'B, R Row Rotations - Real/CORDIC Counter/SR_latch ==
  S : Inport
  R : Inport  Port=2
  AND : Logic  IconShape=distinctive  AllPortsSameDT=off  OutDataTypeStr=boolean
  NOT : Logic  Operator=NOT  IconShape=distinctive  AllPortsSameDT=off  OutDataTypeStr=boolean
  OR : Logic  Operator=OR  IconShape=distinctive  AllPortsSameDT=off  OutDataTypeStr=boolean
  Prev : UnitDelay  InitialCondition=1  SampleTime=-1  HasFrameUpgradeWarning=on
  Q : Outport  VectorParamsAs1DForOutWhenUnconnected=off
  wires:
  S/1 -> OR/1
  OR/1 -> Prev/1
  Prev/1 -> AND/2, Q/1
  AND/1 -> OR/2
  NOT/1 -> AND/1
  R/1 -> NOT/1

== system TxSteering_RxMVDR_4x4_HDL_IQ/DUT/MVDR/Compute Weight Vector/Matrix Left Divide/CORDIC/4x4 Complex CORDIC Matrix Left Divide/Q'B, R 4x4 Complex CORDIC Systolic Array/Leading Complex Row Rotation - 4/Rotate first element to real/Q'B, R Row Rotations - Real/CORDIC Counter/ValidIn to Ready Logic ==
  readyIn : Inport
  validIn : Inport  Port=2
  AND : Logic  IconShape=distinctive  AllPortsSameDT=off  OutDataTypeStr=boolean
  NOT : Logic  Operator=NOT  IconShape=distinctive  AllPortsSameDT=off  OutDataTypeStr=boolean
  readyOut : Outport  VectorParamsAs1DForOutWhenUnconnected=off
  wires:
  validIn/1 -> NOT/1
  readyIn/1 -> AND/1
  AND/1 -> readyOut/1
  NOT/1 -> AND/2

== system TxSteering_RxMVDR_4x4_HDL_IQ/DUT/MVDR/Compute Weight Vector/Matrix Left Divide/CORDIC/4x4 Complex CORDIC Matrix Left Divide/Q'B, R 4x4 Complex CORDIC Systolic Array/Leading Complex Row Rotation - 4/Rotate first element to real - 1/Q'B, R Row Rotations - Real/CORDIC Counter/SR_latch ==
  S : Inport
  R : Inport  Port=2
  AND : Logic  IconShape=distinctive  AllPortsSameDT=off  OutDataTypeStr=boolean
  NOT : Logic  Operator=NOT  IconShape=distinctive  AllPortsSameDT=off  OutDataTypeStr=boolean
  OR : Logic  Operator=OR  IconShape=distinctive  AllPortsSameDT=off  OutDataTypeStr=boolean
  Prev : UnitDelay  InitialCondition=1  SampleTime=-1  HasFrameUpgradeWarning=on
  Q : Outport  VectorParamsAs1DForOutWhenUnconnected=off
  wires:
  R/1 -> NOT/1
  NOT/1 -> AND/1
  AND/1 -> OR/2
  Prev/1 -> Q/1, AND/2
  OR/1 -> Prev/1
  S/1 -> OR/1

== system TxSteering_RxMVDR_4x4_HDL_IQ/DUT/MVDR/Compute Weight Vector/Matrix Left Divide/CORDIC/4x4 Complex CORDIC Matrix Left Divide/Q'B, R 4x4 Complex CORDIC Systolic Array/Leading Complex Row Rotation - 4/Rotate first element to real - 1/Q'B, R Row Rotations - Real/CORDIC Counter/ValidIn to Ready Logic ==
  readyIn : Inport
  validIn : Inport  Port=2
  AND : Logic  IconShape=distinctive  AllPortsSameDT=off  OutDataTypeStr=boolean
  NOT : Logic  Operator=NOT  IconShape=distinctive  AllPortsSameDT=off  OutDataTypeStr=boolean
  readyOut : Outport  VectorParamsAs1DForOutWhenUnconnected=off
  wires:
  validIn/1 -> NOT/1
  readyIn/1 -> AND/1
  AND/1 -> readyOut/1
  NOT/1 -> AND/2
